simulink model "q2"  (R2018a)
settings: Solver=FixedStepAuto  StartTime=0.0  StopTime=0.04  FixedStep=1e-7  RelTol=1e-3
libraries: powerlib x12, simulink x2, powerlib_meascontrol x1
settings Model: Creator=ASUS  LastModifiedBy=ASUS

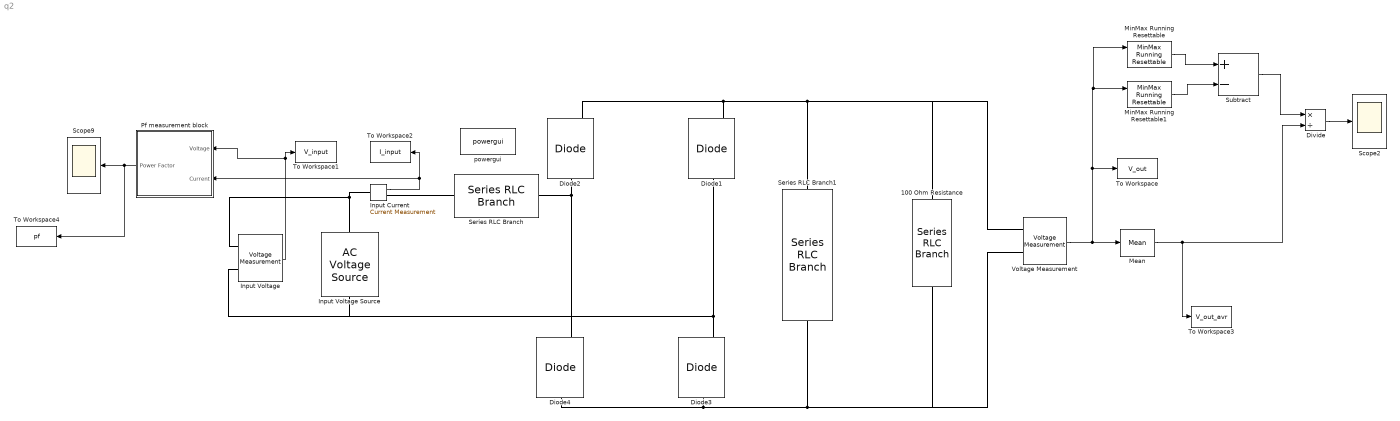
== system q2 ==
  100 Ohm Resistance : powerlib/Elements/Series RLC Branch  LConnTagsString=__new0  RConnTagsString=__new0  BranchType=R  Resistance=100  Inductance=1e-3  SetiL0=off  InitialCurrent=0  Capacitance=1e-6  Setx0=off  InitialVoltage=0  Measurements=None
  Diode{1..4} (4 alike) : powerlib/Power Electronics/Diode  Ron=0.001  Lon=0  Vf=0.8  IC=0  UseSnubber=0  Rs=500  Cs=250e-9  Measurements=on
  Divide : Product  Inputs=*/
  Input Current : powerlib/Measurements/Current Measurement  PhasorSimulation=off  OutputType=Complex  PSBequivalent=0
  Input Voltage : powerlib/Measurements/Voltage Measurement  PhasorSimulation=off  OutputType=Complex  PSBequivalent=0
  Input Voltage Source : powerlib/Electrical Sources/AC Voltage Source  Amplitude=230*sqrt(2)  Phase=0  Frequency=50  SampleTime=0  Measurements=None  BusType=swing  Pref=10e3  Qref=0  Qmin=-inf  Qmax=+inf
  Mean : powerlib_meascontrol/Measurements/Mean  Freq=50  Vinit=0  Ts=0
  MinMax Running Resettable : simulink/Math Operations/MinMax Running Resettable  Function=max  vinit=0
  MinMax Running Resettable1 : simulink/Math Operations/MinMax Running Resettable  Function=min  vinit=900
  "Pf measurement block " : Subsystem
  Scope2 : Scope
  Scope9 : Scope
  Series RLC Branch : powerlib/Elements/Series RLC Branch  LConnTagsString=__new0  RConnTagsString=__new0  BranchType=RL  Resistance=1e-3  Inductance=1e-3  SetiL0=off  InitialCurrent=0  Capacitance=1e-6  Setx0=off  InitialVoltage=0  Measurements=None
  Series RLC Branch1 : powerlib/Elements/Series RLC Branch  LConnTagsString=__new0  RConnTagsString=__new0  BranchType=C  Resistance=1  Inductance=1e-3  SetiL0=off  InitialCurrent=0  Capacitance=19e-4  Setx0=on  InitialVoltage=320  Measurements=None
  Subtract : Sum  Inputs=+-
  To Workspace : ToWorkspace  VariableName=V_out  SaveFormat=Timeseries  SampleTime=-1
  To Workspace1 : ToWorkspace  VariableName=V_input  SaveFormat=Timeseries  SampleTime=-1
  To Workspace2 : ToWorkspace  VariableName=I_input  SaveFormat=Timeseries  SampleTime=-1
  To Workspace3 : ToWorkspace  VariableName=V_out_avr  SaveFormat=Timeseries  SampleTime=-1
  To Workspace4 : ToWorkspace  VariableName=pf  SaveFormat=Timeseries  SampleTime=-1
  Voltage Measurement : powerlib/Measurements/Voltage Measurement  PhasorSimulation=off  OutputType=Complex  PSBequivalent=0
  powergui : powerlib/powergui  Priority=1  SimulationMode=Discrete  SampleTime=50e-6  frequency=60  Iterations=50  frequencyindice=50  Pbase=100e6  ErrMax=1e-4  UnitsV=kV  UnitsW=MW  buscounter=0  FunctionMessages=off  echomessages=off  EnableUseOfTLC=off  CurrentSourceSwitches=off  DisableSnubberDevices=off  DisableRonSwitches=off  DisableVfSwitches=off  DisplayEquations=off  SolverType=Tustin/Backward Euler (TBE)  Interpol=off  ExternalGateDelay=off  methode=off  Ts=100  x0status=blocks  SPID=off  SwTol=0  HookPort=off  RestoreLinks=warning  ResistiveCurrentMeasurement=off  Frange=[0:2:500]  Ylog=off  Xlog=on  ShowGrid=off  save=off  variable=ZData  structure=Input_Current  ZoomFFT=off  StartTime=0.00  cycles=2  DisplayStyle=1  fundamental=50  FreqAxis=off  MaxFrequency=500  frequencyindicesteady=1  RmsSteady=1  display=off
  wires:
  Voltage Measurement/1 -> To Workspace/1, MinMax Running Resettable/1, MinMax Running Resettable1/1, Mean/1
  MinMax Running Resettable/1 -> Subtract/1
  MinMax Running Resettable1/1 -> Subtract/2
  Divide/1 -> Scope2/1
  Subtract/1 -> Divide/1
  Mean/1 -> To Workspace3/1, Divide/2
  Input Voltage/1 -> "Pf measurement block "/1("Voltage "), To Workspace1/1
  Input Current/1 -> "Pf measurement block "/2("Current "), To Workspace2/1
  "Pf measurement block "/1(Power Factor) -> Scope9/1, To Workspace4/1
  connections:
  Input Voltage Source/RConn1 -- Input Current/LConn1 -- Input Voltage/LConn1
  Series RLC Branch/RConn1 -- Diode2/LConn1 -- Diode4/RConn1
  Diode3/RConn1 -- Input Voltage Source/LConn1 -- Input Voltage/LConn2 -- Diode1/LConn1
  Voltage Measurement/LConn2 -- 100 Ohm Resistance/RConn1 -- Series RLC Branch1/RConn1 -- Diode4/LConn1 -- Diode3/LConn1
  Voltage Measurement/LConn1 -- 100 Ohm Resistance/LConn1 -- Series RLC Branch1/LConn1 -- Diode2/RConn1 -- Diode1/RConn1
  Input Current/RConn1 -- Series RLC Branch/LConn1

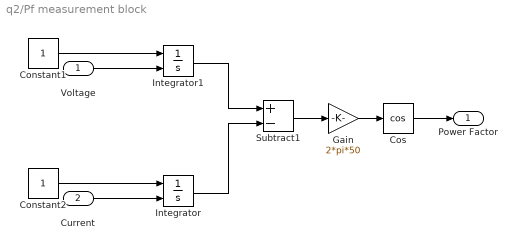
== system q2/Pf measurement block  ==
  "Voltage " : Inport
  "Current " : Inport  Port=2
  Constant1 : Constant
  Constant2 : Constant
  Cos : Trigonometry  Operator=cos
  Gain : Gain  Gain=2*pi*50
  Integrator : Integrator  ExternalReset=falling
  Integrator1 : Integrator  ExternalReset=falling
  Subtract1 : Sum  Inputs=+-
  Power Factor : Outport
  wires:
  Constant2/1 -> Integrator/1
  Cos/1 -> Power Factor/1
  Integrator/1 -> Subtract1/2
  Subtract1/1 -> Gain/1
  "Voltage "/1 -> Integrator1/2
  Gain/1 -> Cos/1
  "Current "/1 -> Integrator/2
  Integrator1/1 -> Subtract1/1
  Constant1/1 -> Integrator1/1
